simulink model "controlSystem_block"  (R2022b)
settings: Solver=VariableStepAuto  StartTime=0.0  StopTime=10.0  RelTol=1e-3
libraries: aerolibanimutils x1
settings Model: Creator=lasto  LastModifiedBy=lasto

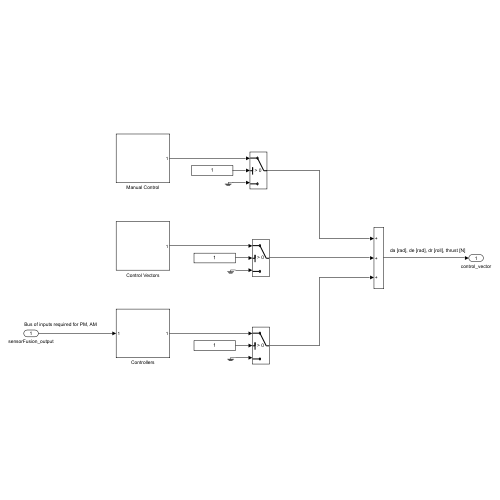
[thumbnail: Simulink's stored preview of the top-level diagram]
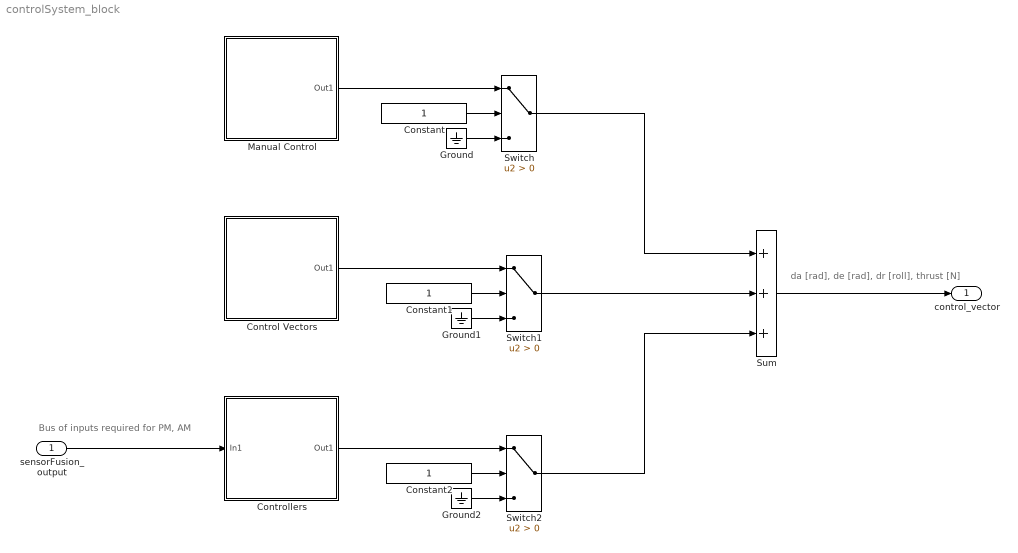
== system controlSystem_block ==
  note: da [rad], de [rad], dr [roll], thrust [N]
  note: Bus of inputs required for PM, AM
  sensorFusion_output : Inport
  Constant : Constant
  Constant1 : Constant
  Constant2 : Constant
  Control Vectors : Subsystem
  Controllers : Subsystem
  Ground : Ground
  Ground1 : Ground
  Ground2 : Ground
  Manual Control : Subsystem
  Sum : Sum  Inputs=+++
  Switch : Switch  Criteria=u2 > Threshold  SaturateOnIntegerOverflow=off  InputSameDT=off
  Switch1 : Switch  Criteria=u2 > Threshold  SaturateOnIntegerOverflow=off  InputSameDT=off
  Switch2 : Switch  Criteria=u2 > Threshold  SaturateOnIntegerOverflow=off  InputSameDT=off
  control_vector : Outport
  wires:
  Switch1/1 -> Sum/2
  Switch2/1 -> Sum/3
  Switch/1 -> Sum/1
  Constant2/1 -> Switch2/2
  Constant/1 -> Switch/2
  Ground1/1 -> Switch1/3
  Sum/1 -> control_vector/1
  Constant1/1 -> Switch1/2
  Ground2/1 -> Switch2/3
  Controllers/1(Out1) -> Switch2/1
  Control Vectors/1(Out1) -> Switch1/1
  Manual Control/1(Out1) -> Switch/1
  Ground/1 -> Switch/3
  sensorFusion_output/1 -> Controllers/1(In1)

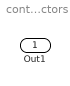
== system controlSystem_block/Control Vectors ==
  Out1 : Outport
  wires:
  ? -> Out1/1

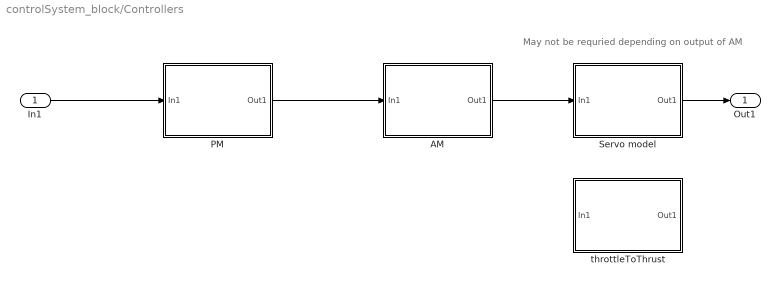
== system controlSystem_block/Controllers ==
  note: May not be requried depending on output of AM
  In1 : Inport
  AM : Subsystem
  PM : Subsystem
  Servo model : Subsystem
  throttleToThrust : Subsystem
  Out1 : Outport
  wires:
  In1/1 -> PM/1(In1)
  PM/1(Out1) -> AM/1(In1)
  AM/1(Out1) -> Servo model/1(In1)
  Servo model/1(Out1) -> Out1/1

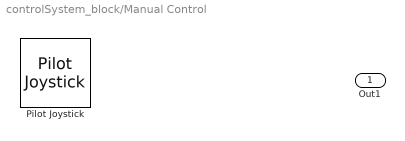
== system controlSystem_block/Manual Control ==
  Pilot Joystick : aerolibanimutils/Pilot Joystick  JoystickID=Joystick1  OutputConfiguration=FourAxis  SampleTime=1/30
  Out1 : Outport

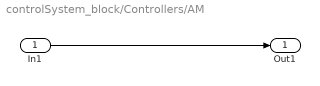
== system controlSystem_block/Controllers/AM ==
  In1 : Inport
  Out1 : Outport
  wires:
  In1/1 -> Out1/1

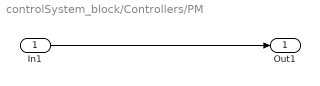
== system controlSystem_block/Controllers/PM ==
  In1 : Inport
  Out1 : Outport
  wires:
  In1/1 -> Out1/1

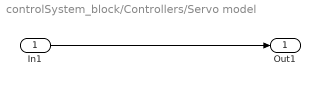
== system controlSystem_block/Controllers/Servo model ==
  In1 : Inport
  Out1 : Outport
  wires:
  In1/1 -> Out1/1

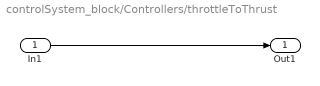
== system controlSystem_block/Controllers/throttleToThrust ==
  In1 : Inport
  Out1 : Outport
  wires:
  In1/1 -> Out1/1
